simulink model "sunlight"  (R2017a)
settings: Solver=FixedStepAuto  StartTime=0.0  StopTime=stoptime  FixedStep=timestep  RelTol=1e-3
undefined symbols (not defined in the file): alpha, fnoise, fseed, omega0, phi0, plo, prx, snoise, tau, timestep
libraries: simulink x2
settings Model: Creator=taehwan  LastModifiedBy=taehwan

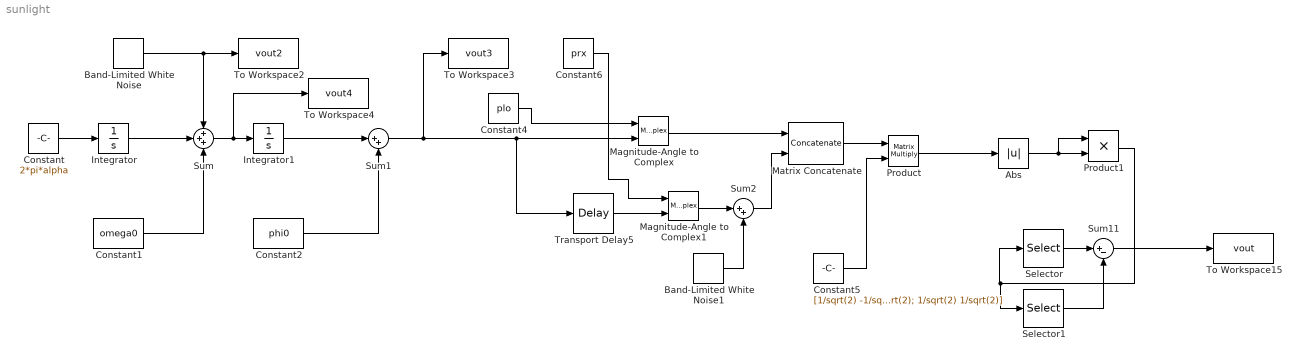
== system sunlight ==
  Abs : Abs
  Band-Limited White Noise : simulink/Sources/Band-Limited White Noise  Cov=[fnoise*2*pi]  Ts=timestep  seed=[fseed]
  Band-Limited White Noise1 : simulink/Sources/Band-Limited White Noise  Cov=2*pi*snoise  Ts=timestep  seed=sseed
  Constant : Constant  Value=2*pi*alpha
  Constant1 : Constant  Value=omega0
  Constant2 : Constant  Value=phi0
  Constant4 : Constant  Value=plo
  Constant5 : Constant  Value=[1/sqrt(2) -1/sqrt(2); 1/sqrt(2) 1/sqrt(2)]
  Constant6 : Constant  Value=prx
  Integrator : Integrator
  Integrator1 : Integrator
  Magnitude-Angle to Complex : MagnitudeAngleToComplex
  Magnitude-Angle to Complex1 : MagnitudeAngleToComplex
  Matrix Concatenate : Concatenate  Mode=Multidimensional array  ConcatenateDimension=2
  Product : Product  Multiplication=Matrix(*)
  Product1 : Product
  Selector : Selector  InputPortWidth=2  IndexOptions=Index vector (dialog)  Indices=[1]  OutputSizes=1
  Selector1 : Selector  InputPortWidth=2  IndexOptions=Index vector (dialog)  Indices=[2]  OutputSizes=1
  Sum : Sum  Inputs=+++
  Sum1 : Sum  Inputs=|++
  Sum11 : Sum  Inputs=|+-
  Sum2 : Sum  Inputs=|++
  To Workspace15 : ToWorkspace  VariableName=vout  SaveFormat=Timeseries  SampleTime=-1
  To Workspace2 : ToWorkspace  VariableName=vout2  SaveFormat=Timeseries  SampleTime=-1
  To Workspace3 : ToWorkspace  VariableName=vout3  SaveFormat=Timeseries  SampleTime=-1
  To Workspace4 : ToWorkspace  VariableName=vout4  SaveFormat=Timeseries  SampleTime=-1
  Transport Delay5 : TransportDelay  DelayTime=tau  BufferSize=2048
  wires:
  Constant/1 -> Integrator/1
  Sum/1 -> To Workspace4/1, Integrator1/1
  Integrator1/1 -> Sum1/1
  Constant2/1 -> Sum1/2
  Sum1/1 -> To Workspace3/1, Transport Delay5/1, Magnitude-Angle to Complex/2
  Constant1/1 -> Sum/3
  Integrator/1 -> Sum/2
  Band-Limited White Noise/1 -> Sum/1, To Workspace2/1
  Magnitude-Angle to Complex/1 -> Matrix Concatenate/1
  Constant4/1 -> Magnitude-Angle to Complex/1
  Constant5/1 -> Product/2
  Transport Delay5/1 -> Magnitude-Angle to Complex1/2
  Matrix Concatenate/1 -> Product/1
  Product/1 -> Abs/1
  Selector/1 -> Sum11/1
  Selector1/1 -> Sum11/2
  Sum11/1 -> To Workspace15/1
  Constant6/1 -> Magnitude-Angle to Complex1/1
  Abs/1 -> Product1/2, Product1/1
  Product1/1 -> Selector1/1, Selector/1
  Band-Limited White Noise1/1 -> Sum2/2
  Magnitude-Angle to Complex1/1 -> Sum2/1
  Sum2/1 -> Matrix Concatenate/2
